simulink model "H175_Stage_01_Anode_Cathode"  (R2023a)
settings: Solver=VariableStepAuto  StartTime=0.0  StopTime=500  RelTol=1e-3
values from neighbouring files (symbols this model uses):
  anode_tube_D = 0.01    [All_Properties.mat]    (also in anode_subsystem_parameters.m; environment_parameters.m)
  D = 0.01    [All_Properties.mat]    (also in anode_subsystem_parameters.m)
  densityHydrogen = 0.0899    [All_Properties.mat]    (also in Valve_Init.m; anode_subsystem_parameters.m)
  Fischer_EMTC120K_supplier_mdot_TLU = [33.385172 57.11265182 82.35238332 173.9183787 230.2050798 50.1655574 86.1774137 122.96585 210.0188714 258.8737112 70.20710678 115.3896052 ... (25 elements, 5x5)]    [All_Properties.mat]    (also in cathode_subsystem_parameters.m = [33.385172 50.1655574 70.20710678 87.4902972 105.3161257)
  Fischer_EMTC120K_supplier_pr_TLU = [2.452176848 3.067593046 4.01020547 5.11549365 6.10066015 2.450765612 3.07166407 4.0616557 5.112468546 6.108742034 2.432340262 3.033516574 ... (25 elements, 5x5)]    [All_Properties.mat]    (also in cathode_subsystem_parameters.m = [2.452176848 2.450765612 2.432340262 2.407245766 2.37067916)
  Kv_VL6112 = 0.8    [All_Properties.mat]    (also in anode_subsystem_parameters.m)
  N2_T = [-56.55 -50 -40 -30 -20 -10 -5 -4 -3 -2 -1 0 ... (52 elements, 1x52)]    [All_Properties.mat]    (also in anode_subsystem_parameters.m = [-56.55 -50 -40 -30 -20 -10 -5 -4 -3 -2 -1 0 1 2 3 4 5 10 20; environment_parameters.m = [-56.55, -50:10:-10, -5:1:5, 10:10:350]; stack_model_harness_parameters.m = [-56.55, -50:10:-10, -5:1:5, 10:10:350])
  p_range = 0.005    [All_Properties.mat]    (also in anode_subsystem_parameters.m)
  r_max = 0.2    [All_Properties.mat]    (also in anode_subsystem_parameters.m)
  r_min = 0.0001    [All_Properties.mat]    (also in anode_subsystem_parameters.m)
  responseTimeValve = 0.013    [All_Properties.mat]    (also in anode_subsystem_parameters.m)
undefined symbols (not defined in the file or in its folder): sigbuilder_block
libraries: fl_lib x168, nesl_utility x116, SimscapeFluids_lib x8, slpidlib x5, simulink x1
(part 8 of 8)

== system H175_Stage_01_Anode_Cathode/Subsystem/ WS6121/Subsystem ==
  Constant : Constant  Value=0
  Liquid water mass flow m_liq_H20 : Product
  Liquid water mole flow n_liq_H2O : Sum  Inputs=-+
  M_H2O : Constant  Value=18.015
  M_H2O g/mol : Constant  Value=18.015
  Max : MinMax  Function=max  Inputs=2
  Mixture mole flow n_tot : Product  Inputs=/*
  PS-Simulink Converter : nesl_utility/PS-Simulink Converter  PhysicalDomain=network_engine_domain  SubClassName=ps_output  LeftPortType=input  RightPortType=output  PseudoPeriodic=off  Frequencies=[]  VectorFormat=inherit  Unit=inherit  AffineConversion=off
  PS-Simulink Converter1 : nesl_utility/PS-Simulink Converter  PhysicalDomain=network_engine_domain  SubClassName=ps_output  LeftPortType=input  RightPortType=output  PseudoPeriodic=off  Frequencies=[]  VectorFormat=inherit  Unit=inherit  AffineConversion=off
  PS-Simulink Converter2 : nesl_utility/PS-Simulink Converter  PhysicalDomain=network_engine_domain  SubClassName=ps_output  LeftPortType=input  RightPortType=output  PseudoPeriodic=off  Frequencies=[]  VectorFormat=inherit  Unit=inherit  AffineConversion=off
  RH : fl_lib/Moist Air/Sensors/Humidity & Trace Gas Sensor (MA)  moisture_on=true  moisture_spec=foundation.enum.moistureSpec.RelativeHumidity  trace_gas_on=false  trace_gas_spec=foundation.enum.trace_gas_spec.mole_fraction
      settings: InternalSimscapePortConfiguration="{\"Bottom\":[],\"Left\":[{\"id\":\"A\",\"label\":\"A\",\"type\":\"foundation.moist_air.moist_air\"}],\"Right\":[{\"id\":\"W\",\"label\":\"W\",\"type\":\"output\"}],\"Top\":[]}"
  Saturated water mole fraction y_w_s : Product  Inputs=/*
  Water mole flow if saturated n_sat_H2O : Product
  g/s : Gain  Gain=1000
  water vapor mole flow n_H2O : Product  Inputs=*/
  y_H2O : fl_lib/Moist Air/Sensors/Humidity & Trace Gas Sensor (MA)  moisture_on=true  moisture_spec=foundation.enum.moistureSpec.MoleFraction  trace_gas_on=false  trace_gas_spec=foundation.enum.trace_gas_spec.mole_fraction
      settings: InternalSimscapePortConfiguration="{\"Bottom\":[],\"Left\":[{\"id\":\"A\",\"label\":\"A\",\"type\":\"foundation.moist_air.moist_air\"}],\"Right\":[{\"id\":\"W\",\"label\":\"W\",\"type\":\"output\"}],\"Top\":[]}"
  rhw : PMIOPort  Side=Left
  mw : PMIOPort  Port=2  Side=Left
  m_liq : Outport
  wires:
  Constant/1 -> Max/1
  Max/1 -> m_liq/1
  water vapor mole flow n_H2O/1 -> Mixture mole flow n_tot/2, Liquid water mole flow n_liq_H2O/2
  PS-Simulink Converter1/1 -> g/s/1
  Liquid water mole flow n_liq_H2O/1 -> Liquid water mass flow m_liq_H20/2
  PS-Simulink Converter/1 -> Saturated water mole fraction y_w_s/1
  Liquid water mass flow m_liq_H20/1 -> Max/2
  Water mole flow if saturated n_sat_H2O/1 -> Liquid water mole flow n_liq_H2O/1
  g/s/1 -> water vapor mole flow n_H2O/1
  Saturated water mole fraction y_w_s/1 -> Water mole flow if saturated n_sat_H2O/1
  PS-Simulink Converter2/1 -> Mixture mole flow n_tot/1, Saturated water mole fraction y_w_s/2
  Mixture mole flow n_tot/1 -> Water mole flow if saturated n_sat_H2O/2
  M_H2O/1 -> Liquid water mass flow m_liq_H20/1
  M_H2O g/mol/1 -> water vapor mole flow n_H2O/2
  connections:
  y_H2O/LConn1 -- rhw/RConn1 -- RH/LConn1
  PS-Simulink Converter2/LConn1 -- y_H2O/RConn1
  PS-Simulink Converter/LConn1 -- RH/RConn1
  mw/RConn1 -- PS-Simulink Converter1/LConn1

== system H175_Stage_01_Anode_Cathode/Subsystem/ WS6121/ValveControl ==
  Simulink-PS Converter1 : nesl_utility/Simulink-PS Converter  PhysicalDomain=network_engine_domain  SubClassName=ps_input  LeftPortType=input  RightPortType=output  PseudoPeriodic=off  Frequencies=[]  NoiseDistribution=none  NoiseParameters=[]  Unit=m^2  AffineConversion=off  FilteringAndDerivatives=provide  SimscapeFilterOrder=1  InputFilterTimeConstant=0.001  UdotUserProvided=0
  Step2 : Step  Time=10  SampleTime=0
  Transfer Fcn2 : TransferFcn  Numerator=[4.75e-6]  Denominator=[1 1]
  Cmd : PMIOPort  Side=Right
  wires:
  Transfer Fcn2/1 -> Simulink-PS Converter1/1
  Step2/1 -> Transfer Fcn2/1
  connections:
  Simulink-PS Converter1/RConn1 -- Cmd/RConn1

== matlab function H175_Stage_01_Anode_Cathode/Cathode_Plant_Sensors/EAC_Theo_Power/MATLAB Function ==
  data: u input; y output; data input
function y = fcn(u, data)

y = (u^data)-1;

== matlab function H175_Stage_01_Anode_Cathode/Cathode_Plant_Sensors/EAT_Theo_Power/MATLAB Function ==
  data: u input; y output; data input
function y = fcn(u, data)

y = (u^data)-1;

== matlab function H175_Stage_01_Anode_Cathode/Anode Controller/APRV_VL6112 Valve_Control/Valve Lift Command Control ==
  data: m_dot input; p1 input; p2 input; T1 input; Kvs input; lift_signal output; rho_std input; W output
function [lift_signal,W]  = fcn(m_dot,p1,p2,T1,Kvs,rho_std)

% calculation based on Bürkert. Direktwirkendes 2-Wege-Standard-Proportionalventil. Datenblatt
% for calculation based on Swagelok. Valve Sizing. Technical Bulletin:
% check calculation_valve_formulas_comparison

% determine optimum valve opening based on pressure ratio for subscritical conditions
% Kvs - valve coefficient [m^3/h] at fully valve open
% lift_signal = Kv/Kvs (linear assumption)

dp = max(0,p1 - p2);            % avoid complex square root

% distinction of flow characteristics based on pressure drop
if p2/p1 > 0.5
    % low pressure drop - subsonic flow
    lift_signal = m_dot*3.6/(Kvs*514)*sqrt(T1/(p2*dp*rho_std));
    W=1;
  
else 
    % high pressure drop - sonic flow (independent of downstream pressure)
    %lift_signal = 0.05;
    lift_signal = m_dot*3.6/(Kvs*257*p1)*sqrt(T1/rho_std);
     W=2;
end
